simulink model "MotorXplorer"  (R2024b)
settings: Solver=FixedStepAuto  StartTime=0.0  StopTime=inf  FixedStep=0.01  RelTol=1e-3
undefined symbols (not defined in the file): Blocking, LF, Non
libraries: hdlsllib x5, amg_usbconverter_n_connect_lib x3
settings Model: Creator=beamk  LastModifiedBy=bpbeam

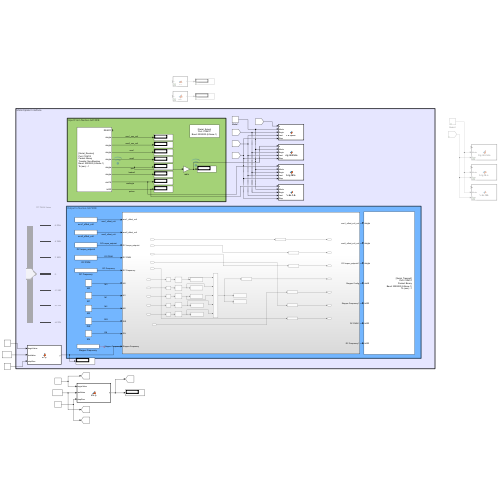
[thumbnail: Simulink's stored preview of the top-level diagram]
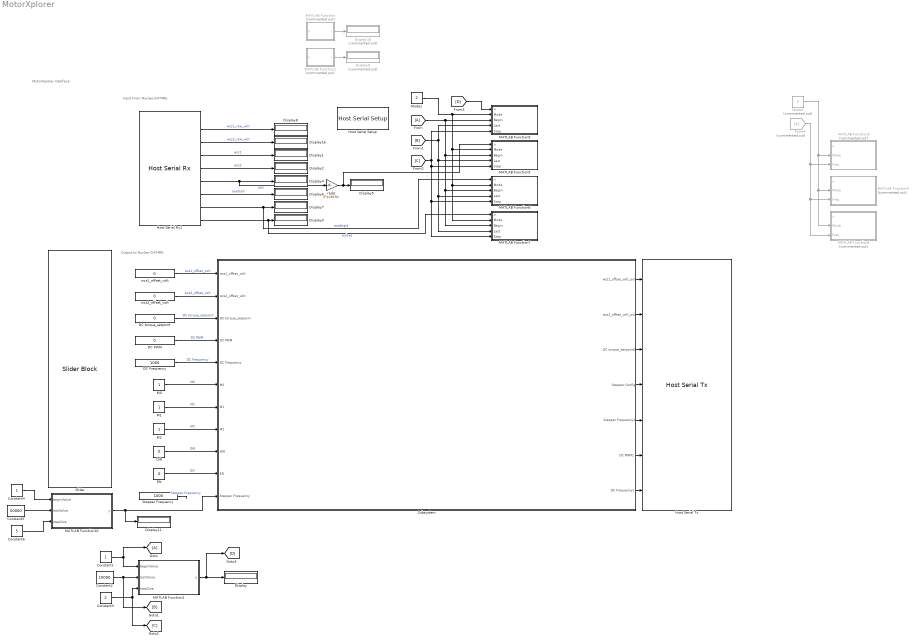
== system MotorXplorer ==
  note: Output to Nucleo-G474RE
  note: Input From Nucleo-G474RE
  note: MotorXploler Interface
  Constant1 : Constant  OutDataTypeStr=int32
  Constant2 : Constant  Value=10000  OutDataTypeStr=int32
  Constant3 : Constant  Value=2  OutDataTypeStr=int32
  Constant4 : Constant  OutDataTypeStr=int32
  Constant5 : Constant  Value=50000  OutDataTypeStr=int32
  Constant6 : Constant  Value=5  OutDataTypeStr=int32
  DC Frequency : Constant  Value=1000
  DC PWM : Constant  Value=0
  DC torque_setpoint : Constant  Value=0
  DIR : Constant  Value=0  OutDataTypeStr=uint8
  Display{,1..8,11,16} (11 alike) : Display
  Display10 : Display  Commented=on
  Display9 : Display  Commented=on
  EN : Constant  Value=0  OutDataTypeStr=uint8
  From : From
  From4 : From  Commented=on
  Goto : Goto
  Host Serial Rx1 : amg_usbconverter_n_connect_lib/Host Serial Rx  conf=rx  port=<auto>  baudrate=2000000  databits=8  parity=None  stopbit=1  flowcontrol=None  transfer=Non-Blocking  timeout=5  packetmode=Binary  enableinitialvalues=off  initialvalues=[]  binheader='45'  binterminator='A'  porttype_double=0  porttype_single=6  porttype_int8=0  porttype_uint8=0  porttype_int16=0  porttype_uint16=1  porttype_int32=1  porttype_uint32=0  asciiformat='%f,%f,%d,%d'  rx_asciiterminator="LF (0x0A - \"\\n\")"  tx_asciiterminator="CRLF (0x0D 0x0A - \"\\r\\n\")"  sampletime=-1  enablecustomportlabel=off  cinputportlabel=0  coutputportlabel=A  portpinstr=0  blockid=HostSerialRx1  inputporttype=[]  inputportwidth=[]  inputportlabel={}  outputporttype=[3 1 1 1 1 1 1 5 6]  outputportwidth=[1 1 1 1 1 1 1 1 1]  outputportlabel={'READY','single','single','single','single','single','single','uint16','int32'}  compat=0  optionstring=[]  autoport='COM12'
  Host Serial Setup : amg_usbconverter_n_connect_lib/Host Serial Setup  conf=setup  port=<auto>  baudrate=2000000  databits=8  parity=None  stopbit=1  flowcontrol=None  transfer=Blocking  timeout=2  packetmode=Binary  initialvalues=[]  binheader='7E 7E'  binterminator='03 03'  porttype_double=0  porttype_single=1  porttype_int8=0  porttype_uint8=0  porttype_int16=0  porttype_uint16=0  porttype_int32=0  porttype_uint32=2  asciiformat='%d %u %x'  rx_asciiterminator="CRLF (0x0D 0x0A - \"\\r\\n\")"  tx_asciiterminator="CRLF (0x0D 0x0A - \"\\r\\n\")"  sampletime=-1  enablecustomportlabel=off  cinputportlabel=0  coutputportlabel=A  portpinstr=0  blockid=HostSerialSetup  inputporttype=[]  inputportwidth=[]  inputportlabel={}  outputporttype=[]  outputportwidth=[]  outputportlabel={}  compat=0  optionstring=[]  autoport='COM12'
  Host Serial Tx : amg_usbconverter_n_connect_lib/Host Serial Tx  conf=tx  port=<auto>  baudrate=2000000  databits=8  parity=None  stopbit=1  flowcontrol=None  transfer=Blocking  timeout=2  packetmode=Binary  initialvalues=[]  binheader='45'  binterminator='A'  porttype_double=0  porttype_single=3  porttype_int8=0  porttype_uint8=1  porttype_int16=0  porttype_uint16=0  porttype_int32=3  porttype_uint32=0  asciiformat='%d,%f'  rx_asciiterminator="CRLF (0x0D 0x0A - \"\\r\\n\")"  tx_asciiterminator="CRLF (0x0D 0x0A - \"\\r\\n\")"  sampletime=-1  enablecustomportlabel=off  cinputportlabel=0  coutputportlabel=A  portpinstr=0  blockid=HostSerialTx  inputporttype=[1 1 1 3 6 6 6]  inputportwidth=[1 1 1 1 1 1 1]  inputportlabel={'single','single','single','uint8','int32','int32','int32'}  outputporttype=[]  outputportwidth=[]  outputportlabel={}  compat=0  optionstring=[]  autoport='COM12'
      settings: SourceProductName=aMG USB Converter N
  M0 : Constant  OutDataTypeStr=uint8
  M1 : Constant  OutDataTypeStr=uint8
  M2 : Constant  OutDataTypeStr=uint8
  MATLAB Function : MATLAB Function  Commented=on  TreatAsAtomicUnit=on
  MATLAB Function1 : MATLAB Function  Commented=on  TreatAsAtomicUnit=on
  MATLAB Function10 : MATLAB Function  TreatAsAtomicUnit=on
  MATLAB Function2 : MATLAB Function  TreatAsAtomicUnit=on
  MATLAB Function3 : MATLAB Function  Commented=on  TreatAsAtomicUnit=on
  MATLAB Function4 : MATLAB Function  Commented=on  TreatAsAtomicUnit=on
  MATLAB Function5 : MATLAB Function  TreatAsAtomicUnit=on
  MATLAB Function6 : MATLAB Function  TreatAsAtomicUnit=on
  MATLAB Function7 : MATLAB Function  TreatAsAtomicUnit=on
  MATLAB Function8 : MATLAB Function  Commented=on  TreatAsAtomicUnit=on
  MATLAB Function9 : MATLAB Function  TreatAsAtomicUnit=on
  Mode1 : Constant  Value=2  OutDataTypeStr=int32
  Mode2 : Constant  Commented=on  Value=2  OutDataTypeStr=int32
  Slider : SliderBlock  ScaleMin=-65535  ScaleMax=65535
  Stepper Frequency : Constant  Value=1000
  Subsystem : Subsystem
  rad/s : Gain  Gain=2*pi/8192
  wcs1_offset_volt : Constant  Value=0  OutDataTypeStr=single
  wcs2_offset_volt : Constant  Value=0  OutDataTypeStr=single
  wires:
  Host Serial Rx1/2 -> Display8/1  "wcs1_raw_volt"
  Host Serial Rx1/3 -> Display16/1  "wcs2_raw_volt"
  Host Serial Rx1/7 -> Display6/1  "loadcell"
  Host Serial Rx1/5 -> Display2/1  "wcs2"
  Host Serial Rx1/6 -> Display4/1, rad/s/1  "pps"
  Host Serial Rx1/4 -> Display1/1  "wcs1"
  wcs1_offset_volt/1 -> Subsystem/1(wcs1_offset_volt)  "wcs1_offset_volt"
  wcs2_offset_volt/1 -> Subsystem/2(wcs2_offset_volt)  "wcs2_offset_volt"
  DC torque_setpoint/1 -> Subsystem/3(DC torque_setpoint)  "DC torque_setpoint"
  DC PWM/1 -> Subsystem/4(DC PWM)  "DC PWM"
  DC Frequency/1 -> Subsystem/5(DC Frequency)  "DC Frequency"
  M0/1 -> Subsystem/6(M0)  "M0"
  M1/1 -> Subsystem/7(M1)  "M1"
  M2/1 -> Subsystem/8(M2)  "M2"
  DIR/1 -> Subsystem/9(DIR)  "DIR"
  EN/1 -> Subsystem/10(EN)  "EN"
  Subsystem/1(wcs1_offset_volt_out) -> Host Serial Tx/1
  Subsystem/2(wcs2_offset_volt_out) -> Host Serial Tx/2
  Subsystem/3(DC torque_setpoint1) -> Host Serial Tx/3
  Subsystem/4(Stepper Config) -> Host Serial Tx/4
  Subsystem/5(Stepper Frequency1) -> Host Serial Tx/5
  Subsystem/6(DC PWM1) -> Host Serial Tx/6
  Subsystem/7(DC Frequency1) -> Host Serial Tx/7
  MATLAB Function/1(i) -> Display10/1
  MATLAB Function1/1(i) -> Display9/1
  Host Serial Rx1/8 -> MATLAB Function6/1(u), Display7/1  "rawAngle"
  rad/s/1 -> MATLAB Function5/1(u), Display5/1
  From/1 -> MATLAB Function9/3(Begin), MATLAB Function5/3(Begin), MATLAB Function7/3(Begin), MATLAB Function6/3(Begin)
  Mode1/1 -> MATLAB Function9/2(Mode), MATLAB Function5/2(Mode), MATLAB Function6/2(Mode), MATLAB Function7/2(Mode)
  Host Serial Rx1/9 -> MATLAB Function7/1(u), Display3/1  "pulses"
  Constant1/1 -> MATLAB Function2/1(beginValue), Goto/1
  Constant2/1 -> MATLAB Function2/2(lastValue), [B]
  Constant3/1 -> MATLAB Function2/3(stepSize), [C]
  MATLAB Function2/1(y) -> [D], Display/1
  [B] -> MATLAB Function9/4(Last), MATLAB Function7/4(Last), MATLAB Function6/4(Last), MATLAB Function5/4(Last)
  [C] -> MATLAB Function9/5(Step), MATLAB Function5/5(Step), MATLAB Function7/5(Step), MATLAB Function6/5(Step)
  [D] -> MATLAB Function9/1(u)
  Mode2/1 -> MATLAB Function8/2(Mode), MATLAB Function4/2(Mode), MATLAB Function3/2(Mode)
  From4/1 -> MATLAB Function8/3(Freq), MATLAB Function4/3(Freq), MATLAB Function3/3(Freq)
  Stepper Frequency/1 -> ?  "Stepper Frequency"
  Constant5/1 -> MATLAB Function10/2(lastValue)
  Constant4/1 -> MATLAB Function10/1(beginValue)
  Constant6/1 -> MATLAB Function10/3(stepSize)
  MATLAB Function10/1(y) -> Display11/1, Subsystem/11(Stepper Frequency)

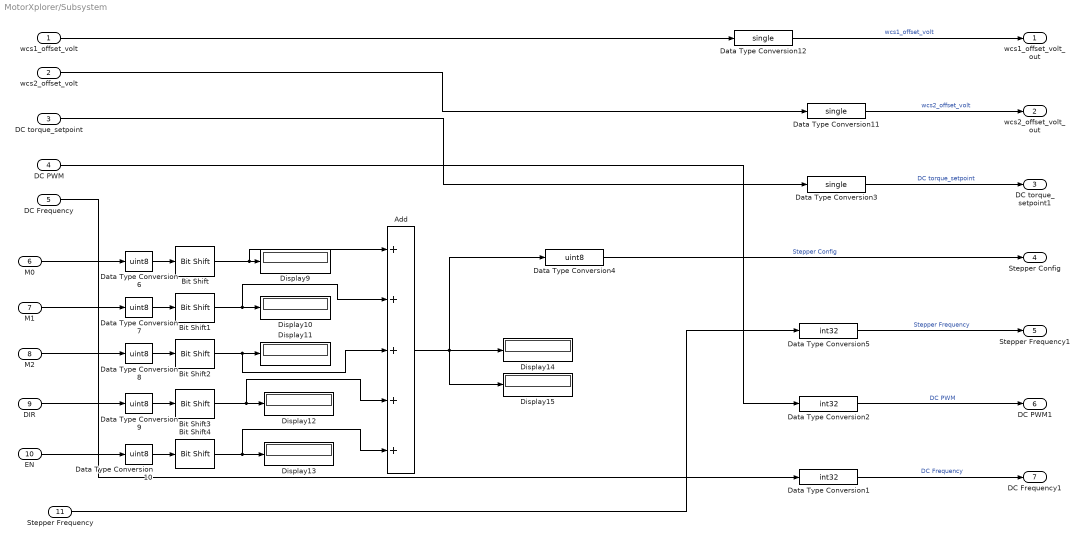
== system MotorXplorer/Subsystem ==
  wcs1_offset_volt : Inport
  wcs2_offset_volt : Inport  Port=2
  DC torque_setpoint : Inport  Port=3
  DC PWM : Inport  Port=4
  DC Frequency : Inport  Port=5
  M0 : Inport  Port=6
  M1 : Inport  Port=7
  M2 : Inport  Port=8
  DIR : Inport  Port=9
  EN : Inport  Port=10
  Stepper Frequency : Inport  Port=11
  Add : Sum  Inputs=+++++
  Bit Shift : hdlsllib/Logic and Bit Operations/Bit Shift  mode=Shift Left Logical  N=4
  Bit Shift1 : hdlsllib/Logic and Bit Operations/Bit Shift  mode=Shift Left Logical  N=3
  Bit Shift2 : hdlsllib/Logic and Bit Operations/Bit Shift  mode=Shift Left Logical  N=2
  Bit Shift3 : hdlsllib/Logic and Bit Operations/Bit Shift  mode=Shift Left Logical  N=1
  Bit Shift4 : hdlsllib/Logic and Bit Operations/Bit Shift  mode=Shift Left Logical  N=0
  Data Type Conversion1 : DataTypeConversion  OutDataTypeStr=int32  SaturateOnIntegerOverflow=off  RndMeth=Floor
  Data Type Conversion{4,6..10} (6 alike) : DataTypeConversion  OutDataTypeStr=uint8  SaturateOnIntegerOverflow=off  RndMeth=Floor
  Data Type Conversion11 : DataTypeConversion  OutDataTypeStr=single  SaturateOnIntegerOverflow=off  RndMeth=Floor
  Data Type Conversion12 : DataTypeConversion  OutDataTypeStr=single  SaturateOnIntegerOverflow=off  RndMeth=Floor
  Data Type Conversion2 : DataTypeConversion  OutDataTypeStr=int32  SaturateOnIntegerOverflow=off  RndMeth=Floor
  Data Type Conversion3 : DataTypeConversion  OutDataTypeStr=single  SaturateOnIntegerOverflow=off  RndMeth=Floor
  Data Type Conversion5 : DataTypeConversion  OutDataTypeStr=int32  SaturateOnIntegerOverflow=off  RndMeth=Floor
  Display{9..15} (7 alike) : Display
      Display10 settings: Format=binary (Stored Integer)
      Display11 settings: Format=binary (Stored Integer)
      Display12 settings: Format=binary (Stored Integer)
      Display13 settings: Format=binary (Stored Integer)
      Display14 settings: Format=binary (Stored Integer)
      Display9 settings: Format=binary (Stored Integer)
  wcs1_offset_volt_out : Outport
  wcs2_offset_volt_out : Outport  Port=2
  DC torque_setpoint1 : Outport  Port=3
  Stepper Config : Outport  Port=4
  Stepper Frequency1 : Outport  Port=5
  DC PWM1 : Outport  Port=6
  DC Frequency1 : Outport  Port=7
  wires:
  Bit Shift/1 -> Display9/1, Add/1
  Data Type Conversion8/1 -> Bit Shift2/1
  EN/1 -> Data Type Conversion10/1
  Data Type Conversion6/1 -> Bit Shift/1
  DC torque_setpoint/1 -> Data Type Conversion3/1
  Data Type Conversion2/1 -> DC PWM1/1  "DC PWM"
  Data Type Conversion7/1 -> Bit Shift1/1
  Data Type Conversion10/1 -> Bit Shift4/1
  DC PWM/1 -> Data Type Conversion2/1
  Bit Shift3/1 -> Display12/1, Add/4
  Data Type Conversion12/1 -> wcs1_offset_volt_out/1  "wcs1_offset_volt"
  Add/1 -> Display15/1, Display14/1, Data Type Conversion4/1
  Bit Shift2/1 -> Display11/1, Add/3
  Stepper Frequency/1 -> Data Type Conversion5/1
  M1/1 -> Data Type Conversion7/1
  Bit Shift1/1 -> Display10/1, Add/2
  Bit Shift4/1 -> Display13/1, Add/5
  M0/1 -> Data Type Conversion6/1
  Data Type Conversion9/1 -> Bit Shift3/1
  Data Type Conversion11/1 -> wcs2_offset_volt_out/1  "wcs2_offset_volt"
  M2/1 -> Data Type Conversion8/1
  wcs1_offset_volt/1 -> Data Type Conversion12/1
  DC Frequency/1 -> Data Type Conversion1/1
  wcs2_offset_volt/1 -> Data Type Conversion11/1
  Data Type Conversion1/1 -> DC Frequency1/1  "DC Frequency"
  DIR/1 -> Data Type Conversion9/1
  Data Type Conversion4/1 -> Stepper Config/1  "Stepper Config"
  Data Type Conversion3/1 -> DC torque_setpoint1/1  "DC torque_setpoint"
  Data Type Conversion5/1 -> Stepper Frequency1/1  "Stepper Frequency"

== matlab function MotorXplorer/MATLAB Function1 ==
  data: v input; i output
function i = fcn(v)

% i = 18.450040563529175 * (v - 0.43) - 30.484959796035263;
i = 14.985111513990505 * (v - 0.454) - 24.732609324758744;

== matlab function MotorXplorer/MATLAB Function ==
  data: v input; i output
function i = fcn(v)

% i = 17.634838383843903 * (v - 0.385) - 29.14389133426229;
i = 14.546740025512696 * (v - 0.395) - 24.036602719877;

== matlab function MotorXplorer/MATLAB Function2 ==
  data: beginValue input; lastValue input; stepSize input; y output
function y = step(beginValue, lastValue, stepSize)
    % Use a persistent variable to store the current value between calls
    persistent currentValue;

    % Initialize the current value on the first function call
    if isempty(currentValue)
        currentValue = beginValue;
    end

    % Check if the current value exceeds the last value
    if currentValue < lastValue
        currentValue = currentValue + stepSize;
    end

    % Output the current value
    y = currentValue;
end

== matlab function MotorXplorer/MATLAB Function3 ==
  data: u input; Mode input; Freq input
function AngVeloData(u, Mode, Freq)
    % Convert Mode and Freq to strings for the variable name
    varName = sprintf('AngVelo_%d_%d', Mode, Freq);

    % Persistent variable to store the data
    persistent data;
    if isempty(data)
        data = [];
    end

    % Append new data
    data = [data; u];

    if size(data, 1) > 1000
        data(1, :) = []; % Remove oldest data if exceeding the limit
    end

    % Export data to the workspace with dynamic variable name
    assignin('base', varName, data);
end

== matlab function MotorXplorer/MATLAB Function4 ==
  data: u input; Mode input; Freq input
function AngData(u, Mode, Freq)
    % u is the input signal
    % Mode and Freq are constant inputs used to name the workspace variable

    % Convert Mode and Freq to strings for the variable name
    varName = sprintf('Ang_%d_%d', Mode, Freq);

    % Persistent variable to store the data
    persistent data;
    if isempty(data)
        data = [];
    end

    % Append new data
    data = [data; u];

    % Limit size of data (optional, for example, 1000 rows)
    % if size(data, 1) > 100000
    %     data(1, :) = []; % Remove oldest data if exceeding the limit
    % end

    % Export data to the workspace with dynamic variable name
    assignin('base', varName, data);
end

== matlab function MotorXplorer/MATLAB Function5 ==
  data: u input; Mode input; Begin input; Last input; Step input
function AngVeloData(u, Mode, Begin, Last, Step)
    % u is the input signal
    % Mode and Freq are constant inputs used to name the workspace variable

    % Convert Mode and Freq to strings for the variable name
    varName = sprintf('AngVelo_%d_%d_%d_%d', Mode, Begin, Last, Step);

    % Persistent variable to store the data
    persistent data;
    if isempty(data)
        data = [];
    end

    % Append new data
    data = [data; u];

    % Export data to the workspace with dynamic variable name
    assignin('base', varName, data);
end

== matlab function MotorXplorer/MATLAB Function6 ==
  data: u input; Mode input; Begin input; Last input; Step input
function AngData(u, Mode, Begin, Last, Step)
    % u is the input signal
    % Mode and Freq are constant inputs used to name the workspace variable

    % Convert Mode and Freq to strings for the variable name
    varName = sprintf('Ang_%d_%d_%d_%d', Mode, Begin, Last, Step);

    % Persistent variable to store the data
    persistent data;
    if isempty(data)
        data = [];
    end

    % Append new data
    data = [data; u];

    % Export data to the workspace with dynamic variable name
    assignin('base', varName, data);
end

== matlab function MotorXplorer/MATLAB Function7 ==
  data: u input; Mode input; Begin input; Last input; Step input
function PulseData(u, Mode, Begin, Last, Step)
    % u is the input signal
    % Mode and Freq are constant inputs used to name the workspace variable

    % Convert Mode and Freq to strings for the variable name
    varName = sprintf('Pulse_%d_%d_%d_%d', Mode, Begin, Last, Step);

    % Persistent variable to store the data
    persistent data;
    if isempty(data)
        data = [];
    end

    % Append new data
    data = [data; u];

    % Export data to the workspace with dynamic variable name
    assignin('base', varName, data);
end

== matlab function MotorXplorer/MATLAB Function8 ==
  data: u input; Mode input; Freq input
function PulseData(u, Mode, Freq)
    % u is the input signal
    % Mode and Freq are constant inputs used to name the workspace variable

    % Convert Mode and Freq to strings for the variable name
    varName = sprintf('Pulse_%d_%d', Mode, Freq);

    % Persistent variable to store the data
    persistent data;
    if isempty(data)
        data = [];
    end

    % Append new data
    data = [data; u];

    % Limit size of data (optional, for example, 1000 rows)
    % if size(data, 1) > 1000
    %     data(1, :) = []; % Remove oldest data if exceeding the limit
    % end

    % Export data to the workspace with dynamic variable name
    assignin('base', varName, data);
end

== matlab function MotorXplorer/MATLAB Function9 ==
  data: u input; Mode input; Begin input; Last input; Step input
function FreqData(u, Mode, Begin, Last, Step)
    % Convert Mode and Freq to strings for the variable name
    varName = sprintf('Freq_%d_%d_%d_%d', Mode, Begin, Last, Step);

    % Persistent variable to store the data
    persistent data;
    if isempty(data)
        data = [];
    end

    % Append new data
    data = [data; u];

    % Export data to the workspace with dynamic variable name
    assignin('base', varName, data);
end

== matlab function MotorXplorer/MATLAB Function10 ==
  data: beginValue input; lastValue input; stepSize input; y output
function y = step(beginValue, lastValue, stepSize)
    % Use a persistent variable to store the current value between calls
    persistent currentValue;

    % Initialize the current value on the first function call
    if isempty(currentValue)
        currentValue = beginValue;
    end

    % Check if the current value exceeds the last value
    if currentValue > lastValue
        currentValue = currentValue + 0;
    else
        currentValue = currentValue + stepSize;
    end

    % Output the current value
    y = currentValue;
end
